simulink subsystem "SignalProcessing"  (R2023b)
settings: Solver=VariableStepAuto  StartTime=0.0  StopTime=10.0  RelTol=1e-3
undefined symbols (not defined in the file): MCU_Ts
settings Model: DataDictionary=neck_mk3.sldd  EnableAccessToBaseWorkspace=off  Creator=upattacini  LastModifiedBy=upattacini

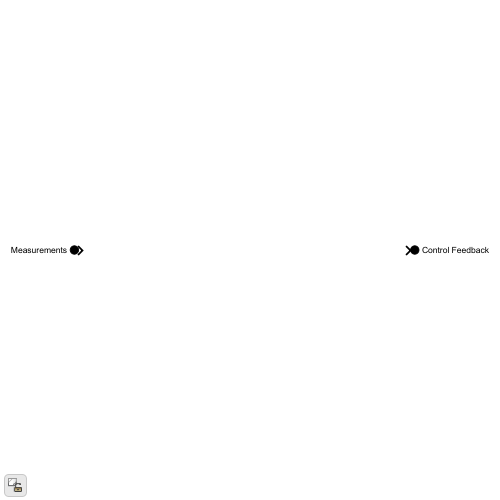
[thumbnail: Simulink's stored preview of the top-level diagram]
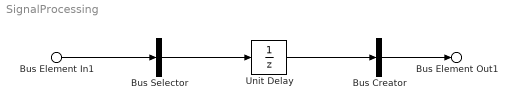
== system SignalProcessing ==
  Bus Element In1 : Inport  PortName=Measurements
  Bus Creator : BusCreator  Inputs=1  OutDataTypeStr=Bus: Data_ControlFeedback  NonVirtualBus=on
      settings: InheritFromInputs=off
  Bus Selector : BusSelector  OutputSignals=Encoders  OutputAsBus=on
  Unit Delay : UnitDelay  SampleTime=MCU_Ts  HasFrameUpgradeWarning=on
  Bus Element Out1 : Outport  PortName=Control Feedback
  wires:
  Unit Delay/1 -> Bus Creator/1
  Bus Element In1/1 -> Bus Selector/1
  Bus Selector/1 -> Unit Delay/1
  Bus Creator/1 -> Bus Element Out1/1
